simulink model "LDPC_Decoder_Ex1"  (R2024a)
settings: Solver=VariableStepAuto  StartTime=0.0  StopTime=64800+64800  RelTol=1e-3
undefined symbols (not defined in the file or in its folder): Configured, DVB, es1, F, Initialized_retain_I, Pre, S, S2, vsva2488, X, xcvr1602
libraries: hdlBasic x37, dspsrcs4 x3, hdlDSPIP x1, vmcUtilities x1
settings Model: Creator=nanumolu  LastModifiedBy=sdegala
settings ConfigComp: CovBoundaryAbsTol=1.0e-5

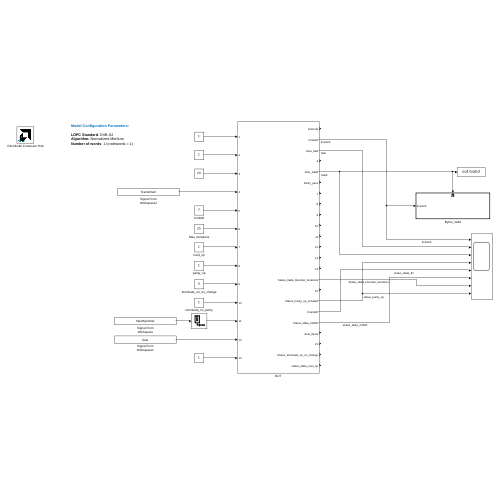
[thumbnail: Simulink's stored preview of the top-level diagram]
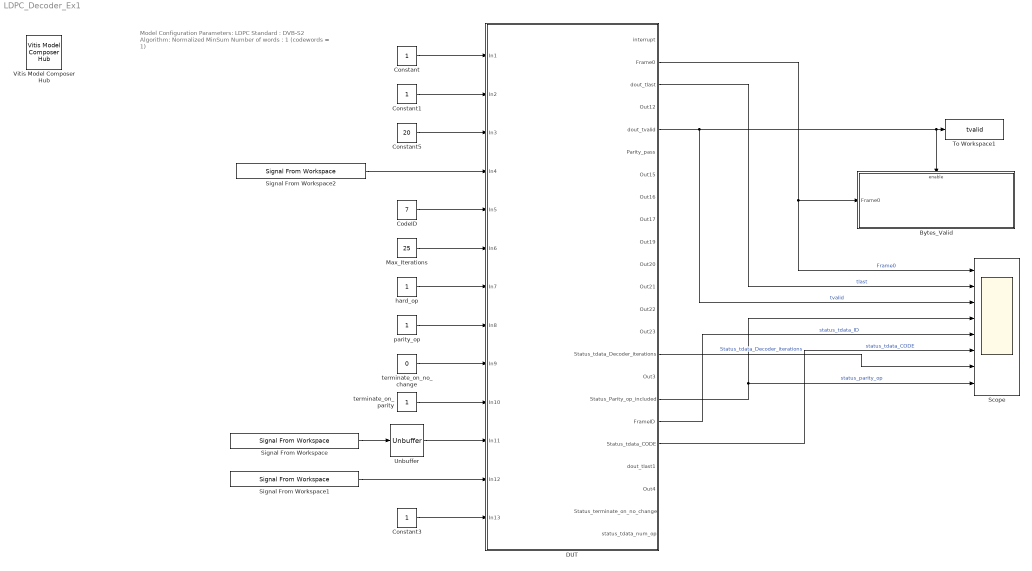
== system LDPC_Decoder_Ex1 ==
  note: Model Configuration Parameters:
      |
      | LDPC Standard : DVB-S2
      | Algorithm: Normalized MinSum
      | Number of words : 1 (codewords = 1)
  Bytes_Valid : Subsystem
  CodeID : Constant  Value=7  SampleTime=1
  Constant : Constant  SampleTime=1
  Constant1 : Constant  SampleTime=1
  Constant3 : Constant  SampleTime=1
  Constant5 : Constant  Value=20  SampleTime=1
  DUT : Subsystem
  Max_Iterations : Constant  Value=25  SampleTime=1
  Scope : Scope  NumInputPorts=8
  Signal From Workspace : dspsrcs4/Signal From Workspace  X=InputSymbols  Ts=1  nsamps=64800  OutputAfterFinalValue=Setting to zero  ignoreOrWarnInputAndFrameLengths=off  OutputFrames=off
  Signal From Workspace1 : dspsrcs4/Signal From Workspace  X=tlast  Ts=1  nsamps=1  OutputAfterFinalValue=Setting to zero  ignoreOrWarnInputAndFrameLengths=off  OutputFrames=off
  Signal From Workspace2 : dspsrcs4/Signal From Workspace  X=FrameNum  Ts=1  nsamps=1  OutputAfterFinalValue=Setting to zero  ignoreOrWarnInputAndFrameLengths=off  OutputFrames=off
  To Workspace1 : ToWorkspace  VariableName=tvalid  SampleTime=-1
      settings: Save2DSignal=2-D array (concatenate along first dimension)
  Unbuffer : Unbuffer
  Vitis Model Composer Hub : vmcUtilities/Vitis Model Composer Hub  Tag=genX  CodeGeneration=off  SubsystemName=DUT  BlockHierPath=Channalizer_smoke  CompilationType=HDLCompilation  SubsystemType=HDLNode  ExportTypeV2=HDL Netlist  StartColumn=1  NumberOfColumns=1  TargetDirectory=./netlist_chan_vlg  exportDesign=on  analyzeDesign=off  validateDesignOnHw=off  ExportType=AI Engines  IpVendor=xilinx.com  IpLibrary=hls  IpVersion=1.0  IpHWLanguage=Verilog  AieCompilerOptions={}  AieSimulatorOptions={}  CreateTestbench=on  TestbenchStackSize=10  RunRtlSim=off  RunCSim=off  RunAieSim=off  AieSimTimeout=50000  RunAieSimProfiling=off  LaunchVitisAnalyzer=off  PlotOutput=off  RunX86Sim=off  X86SimTimeout=10  GenHwImage=off  GenLibadfXo=on  GenHwValidationCode=off  PlatformType=Not Specified  HwSystemType=Baremetal  HwValidationTarget=hw  ProjDevice=xcvr1602-vsva2488-2MP-e-S-es1  ProjDevicePart=xcvr1602-vsva2488-2MP-e-S-es1  AIEType=AIE  SamplePeriod=-1  ClockFrequency=200  DataPathParallelism=1  xilinxfamily=versalairfes1  part=xcvr1602  speed=-2MP-e-S-es1  package=vsva2488  directory=./netlist/ip/DUT/src  testbench=off  incr_netlist=off  synthesis_tool=Vivado  clock_wrapper=Clock Enables  dbl_ovrd=According to Block Masks  dcm_input_clock_period=10  sysclk_period=10  simulink_period=1  eval_field=0  IPInfoJsonString="{\"DUTSubsystemName\":\"Channalizer_smoke\",\"HDLSubsystem\":{\"SubsystemName\":\"Channalizer_smoke\",\"IPName\":\"Copy_of_hamilton_vrf_fft\",\"IPLibrary\":\"VMC\",\"IPVendor\":\"User Company\",\"IPVersion\":\"1.0\",\"TargetDirectory\":\"./netlist_chan_vlg\",\"SubsystemDir\":\"./netlist_chan_vlg/ip/Channalizer_smoke\",\"FreqHz\":\"100000000\"},\"SubsystemTag\":\"HDLNode\"}"  LogFileName=/proj/dsv_xhd/ravalib/Head/Tests/REL/2025.1/dsv/modelcomposer/hdl/regression/channelizer/smoke/netlist_chan_vlg/model_composer.log  NThreads=4  IPConfigFile=/tmp/vmctmp-10364637636032824832/Channalizer_smoke_ipconfig.json
  hard_op : Constant  SampleTime=1
  parity_op : Constant  SampleTime=1
  terminate_on_no_change : Constant  Value=0  SampleTime=1
  terminate_on_parity : Constant  SampleTime=1
  wires:
  Constant/1 -> DUT/1(In1)
  Constant1/1 -> DUT/2(In2)
  Constant5/1 -> DUT/3(In3)
  Signal From Workspace2/1 -> DUT/4(In4)
  CodeID/1 -> DUT/5(In5)
  Max_Iterations/1 -> DUT/6(In6)
  hard_op/1 -> DUT/7(In7)
  parity_op/1 -> DUT/8(In8)
  terminate_on_no_change/1 -> DUT/9(In9)
  terminate_on_parity/1 -> DUT/10(In10)
  Constant3/1 -> DUT/13(In13)
  Signal From Workspace1/1 -> DUT/12(In12)
  DUT/2(Frame0) -> Scope/1, Bytes_Valid/1(Frame0)  "Frame0"
  DUT/5(dout_tvalid) -> To Workspace1/1, Bytes_Valid/Enable, Scope/3  "tvalid"
  DUT/3(dout_tlast) -> Scope/2  "tlast"
  DUT/17(Status_Parity_op_included) -> Scope/4, Scope/8  "status_parity_op"
  DUT/18(FrameID) -> Scope/5  "status_tdata_ID"
  DUT/19(Status_tdata_CODE) -> Scope/6  "status_tdata_CODE"
  Signal From Workspace/1 -> Unbuffer/1
  Unbuffer/1 -> DUT/11(In11)
  DUT/15(Status_tdata_Decoder_iterations) -> Scope/7  "Status_tdata_Decoder_iterations"

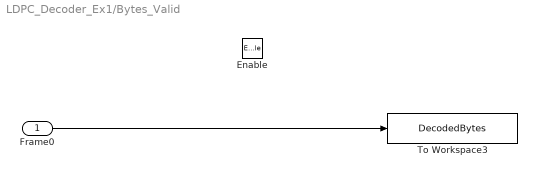
== system LDPC_Decoder_Ex1/Bytes_Valid ==
  Frame0 : Inport
  Enable : EnablePort
  To Workspace3 : ToWorkspace  VariableName=DecodedBytes  SampleTime=-1
      settings: Save2DSignal=2-D array (concatenate along first dimension)
  wires:
  Frame0/1 -> To Workspace3/1

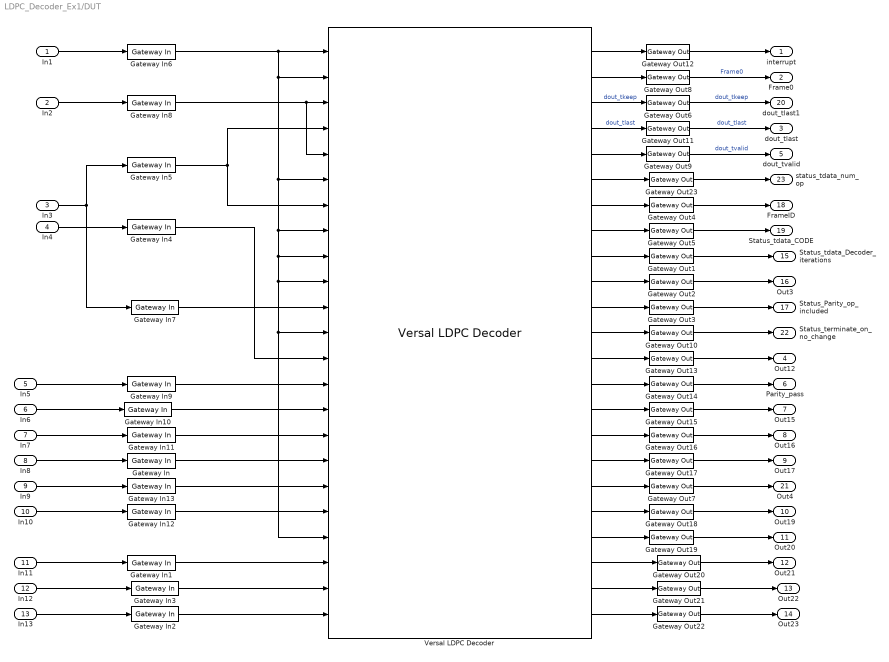
== system LDPC_Decoder_Ex1/DUT ==
  In1 : Inport
  In2 : Inport  Port=2
  In3 : Inport  Port=3
  In4 : Inport  Port=4
  In5 : Inport  Port=5
  In6 : Inport  Port=6
  In7 : Inport  Port=7
  In8 : Inport  Port=8
  In9 : Inport  Port=9
  In10 : Inport  Port=10
  In11 : Inport  Port=11
  In12 : Inport  Port=12
  In13 : Inport  Port=13
  Gateway In{,11..13} (4 alike) : hdlBasic/Gateway In  gui_display_data_type=Fixed-point  arith_type=Unsigned  n_bits=1  bin_pt=0  preci_type=Single  exp_width=8  frac_width=24  rows=1  columns=1  quantization="Round  (unbiased: +/- Inf)"  overflow=Saturate  period=1  UseAsADC=off  ADCChannel='1'  interface=None  automatic_assignment=on  address_offset=hex2dec('00')  intf_name=''  intf_description=''  default_value=0  timing_constraint=None  locs_specified=off  LOCs={}  io_standard={}  inherit_from_input=off  hdl_port=on  XmcBlockStatus=1  maskContainerNames=group4  block_type=gatewayin  block_config=sysgen:gateway_in_config  block_width_w=590  block_height_w=620  block_width=640  block_height=850
  Gateway In1 : hdlBasic/Gateway In  gui_display_data_type=Fixed-point  arith_type=Signed (2's comp)  n_bits=8  bin_pt=2  preci_type=Single  exp_width=8  frac_width=24  rows=1  columns=1  quantization="Round  (unbiased: +/- Inf)"  overflow=Saturate  period=1  UseAsADC=off  ADCChannel='1'  interface=None  automatic_assignment=on  address_offset=hex2dec('00')  intf_name=''  intf_description=''  default_value=0  timing_constraint=None  locs_specified=off  LOCs={}  io_standard={}  inherit_from_input=off  hdl_port=on  XmcBlockStatus=1  maskContainerNames=group4  block_type=gatewayin  block_config=sysgen:gateway_in_config  block_width_w=590  block_height_w=620  block_width=640  block_height=850
  Gateway In10 : hdlBasic/Gateway In  gui_display_data_type=Fixed-point  arith_type=Unsigned  n_bits=6  bin_pt=0  preci_type=Single  exp_width=8  frac_width=24  rows=1  columns=1  quantization="Round  (unbiased: +/- Inf)"  overflow=Saturate  period=1  UseAsADC=off  ADCChannel='1'  interface=None  automatic_assignment=on  address_offset=hex2dec('00')  intf_name=''  intf_description=''  default_value=0  timing_constraint=None  locs_specified=off  LOCs={}  io_standard={}  inherit_from_input=off  hdl_port=on  XmcBlockStatus=1  maskContainerNames=group4  block_type=gatewayin  block_config=sysgen:gateway_in_config  block_width_w=590  block_height_w=620  block_width=640  block_height=850
  Gateway In2 : hdlBasic/Gateway In  gui_display_data_type=Boolean  arith_type=Boolean  n_bits=1  bin_pt=0  preci_type=Single  exp_width=8  frac_width=24  rows=1  columns=1  quantization="Round  (unbiased: +/- Inf)"  overflow=Saturate  period=1  UseAsADC=off  ADCChannel='1'  interface=None  automatic_assignment=on  address_offset=hex2dec('00')  intf_name=''  intf_description=''  default_value=0  timing_constraint=None  locs_specified=off  LOCs={}  io_standard={}  inherit_from_input=off  hdl_port=on  XmcBlockStatus=1  maskContainerNames=group4  block_type=gatewayin  block_config=sysgen:gateway_in_config  block_width_w=590  block_height_w=620  block_width=640  block_height=850
  Gateway In3 : hdlBasic/Gateway In  gui_display_data_type=Boolean  arith_type=Boolean  n_bits=1  bin_pt=0  preci_type=Single  exp_width=8  frac_width=24  rows=1  columns=1  quantization="Round  (unbiased: +/- Inf)"  overflow=Saturate  period=1  UseAsADC=off  ADCChannel='1'  interface=None  automatic_assignment=on  address_offset=hex2dec('00')  intf_name=''  intf_description=''  default_value=0  timing_constraint=None  locs_specified=off  LOCs={}  io_standard={}  inherit_from_input=off  hdl_port=on  XmcBlockStatus=1  maskContainerNames=group4  block_type=gatewayin  block_config=sysgen:gateway_in_config  block_width_w=590  block_height_w=620  block_width=640  block_height=850
  Gateway In4 : hdlBasic/Gateway In  gui_display_data_type=Fixed-point  arith_type=Unsigned  n_bits=8  bin_pt=0  preci_type=Single  exp_width=8  frac_width=24  rows=1  columns=1  quantization="Round  (unbiased: +/- Inf)"  overflow=Saturate  period=1  UseAsADC=off  ADCChannel='1'  interface=None  automatic_assignment=on  address_offset=hex2dec('00')  intf_name=''  intf_description=''  default_value=0  timing_constraint=None  locs_specified=off  LOCs={}  io_standard={}  inherit_from_input=off  hdl_port=on  XmcBlockStatus=1  maskContainerNames=group4  block_type=gatewayin  block_config=sysgen:gateway_in_config  block_width_w=590  block_height_w=620  block_width=640  block_height=850
  Gateway In5 : hdlBasic/Gateway In  gui_display_data_type=Fixed-point  arith_type=Signed (2's comp)  n_bits=18  bin_pt=0  preci_type=Single  exp_width=8  frac_width=24  rows=1  columns=1  quantization="Round  (unbiased: +/- Inf)"  overflow=Saturate  period=1  UseAsADC=off  ADCChannel='1'  interface=None  automatic_assignment=on  address_offset=hex2dec('00')  intf_name=''  intf_description=''  default_value=0  timing_constraint=None  locs_specified=off  LOCs={}  io_standard={}  inherit_from_input=off  hdl_port=on  XmcBlockStatus=1  maskContainerNames=group4  block_type=gatewayin  block_config=sysgen:gateway_in_config  block_width_w=590  block_height_w=620  block_width=640  block_height=850
  Gateway In6 : hdlBasic/Gateway In  gui_display_data_type=Boolean  arith_type=Boolean  n_bits=16  bin_pt=14  preci_type=Single  exp_width=8  frac_width=24  rows=1  columns=1  quantization="Round  (unbiased: +/- Inf)"  overflow=Saturate  period=1  UseAsADC=off  ADCChannel='1'  interface=None  automatic_assignment=on  address_offset=hex2dec('00')  intf_name=''  intf_description=''  default_value=0  timing_constraint=None  locs_specified=off  LOCs={}  io_standard={}  inherit_from_input=off  hdl_port=on  XmcBlockStatus=1  maskContainerNames=group4  block_type=gatewayin  block_config=sysgen:gateway_in_config  block_width_w=590  block_height_w=620  block_width=640  block_height=850
  Gateway In7 : hdlBasic/Gateway In  gui_display_data_type=Fixed-point  arith_type=Signed (2's comp)  n_bits=32  bin_pt=0  preci_type=Single  exp_width=8  frac_width=24  rows=1  columns=1  quantization="Round  (unbiased: +/- Inf)"  overflow=Saturate  period=1  UseAsADC=off  ADCChannel='1'  interface=None  automatic_assignment=on  address_offset=hex2dec('00')  intf_name=''  intf_description=''  default_value=0  timing_constraint=None  locs_specified=off  LOCs={}  io_standard={}  inherit_from_input=off  hdl_port=on  XmcBlockStatus=1  maskContainerNames=group4  block_type=gatewayin  block_config=sysgen:gateway_in_config  block_width_w=590  block_height_w=620  block_width=640  block_height=850
  Gateway In8 : hdlBasic/Gateway In  gui_display_data_type=Boolean  arith_type=Boolean  n_bits=16  bin_pt=14  preci_type=Single  exp_width=8  frac_width=24  rows=1  columns=1  quantization="Round  (unbiased: +/- Inf)"  overflow=Saturate  period=1  UseAsADC=off  ADCChannel='1'  interface=None  automatic_assignment=on  address_offset=hex2dec('00')  intf_name=''  intf_description=''  default_value=0  timing_constraint=None  locs_specified=off  LOCs={}  io_standard={}  inherit_from_input=off  hdl_port=on  XmcBlockStatus=1  maskContainerNames=group4  block_type=gatewayin  block_config=sysgen:gateway_in_config  block_width_w=590  block_height_w=620  block_width=640  block_height=850
  Gateway In9 : hdlBasic/Gateway In  gui_display_data_type=Fixed-point  arith_type=Unsigned  n_bits=7  bin_pt=0  preci_type=Single  exp_width=8  frac_width=24  rows=1  columns=1  quantization="Round  (unbiased: +/- Inf)"  overflow=Saturate  period=1  UseAsADC=off  ADCChannel='1'  interface=None  automatic_assignment=on  address_offset=hex2dec('00')  intf_name=''  intf_description=''  default_value=0  timing_constraint=None  locs_specified=off  LOCs={}  io_standard={}  inherit_from_input=off  hdl_port=on  XmcBlockStatus=1  maskContainerNames=group4  block_type=gatewayin  block_config=sysgen:gateway_in_config  block_width_w=590  block_height_w=620  block_width=640  block_height=850
  Gateway Out{1..7,9..23} (22 alike) : hdlBasic/Gateway Out  inherit_from_input=off  bool_to_boolean=off  hdl_port=on  rows=1  columns=1  UseAsDAC=off  DACChannel='1'  interface=None  automatic_assignment=on  address_offset=hex2dec('00')  intf_name=''  intf_description=''  timing_constraint=None  locs_specified=off  LOCs={}  io_standard={}  XmcBlockStatus=1  maskContainerNames=group4  block_type=gatewayout  block_config=sysgen:gateway_out_config  block_width_w=590  block_height_w=620  block_width=620  block_height=750
  Gateway Out8 : hdlBasic/Gateway Out  inherit_from_input=on  bool_to_boolean=off  hdl_port=on  rows=1  columns=1  UseAsDAC=off  DACChannel='1'  interface=None  automatic_assignment=on  address_offset=hex2dec('00')  intf_name=''  intf_description=''  timing_constraint=None  locs_specified=off  LOCs={}  io_standard={}  XmcBlockStatus=1  maskContainerNames=group4  block_type=gatewayout  block_config=sysgen:gateway_out_config  block_width_w=590  block_height_w=620  block_width=620  block_height=750
  Versal LDPC Decoder : hdlDSPIP/Versal LDPC Decoder  standard=DVB-S2(X)  ldpc_decode_algorithm_source=Initialized  ldpc_decode_algorithm_modifier_source=Initialized  ldpc_decode_sat_bits_source=Initialized  ldpc_decode_max_schedule_source=Initialized  ldpc_decode_code_definition='no_file_loaded'  ldpc_decode_overrides=on  ldpc_decode_algorithm=Normalized_MinSum  ldpc_decode_algorithm_modifier=1  ldpc_decode_sat_bits=6B  ldpc_decode_max_schedule=0  parameter_interface=Initialized_retain_I/F  enable_ifs=on  Interrupts=on  ecc_interrupts=None  bypass=off  din_interface=Pre-Configured  din_lanes=1  din_words_configuration=Fixed  din_words=1  dout_interface=Pre-Configured  dout_lanes=1  dout_words_configuration=Fixed  dout_words=1  throughput_utilization=100  ip_name=Versal LDPC Decoder  ip_version=1.0  dsptool_ready=false  ipcore_usecache=true  ipcore_useipmodelcache=true  wrapper_available=true  port_translation_map={ 'aclken' => 'en', aresetn' => 'rst' }  structural_sim=true  ipcore_do_not_force_period=true  XmcBlockStatus=1  maskContainerNames=tabcontainer1  block_type=versal_ldpc_v1_0  block_config=sysgen:rodinimport_config
  interrupt : Outport
  Frame0 : Outport  Port=2
  dout_tlast : Outport  Port=3
  Out12 : Outport  Port=4
  dout_tvalid : Outport  Port=5
  Parity_pass : Outport  Port=6
  Out15 : Outport  Port=7
  Out16 : Outport  Port=8
  Out17 : Outport  Port=9
  Out19 : Outport  Port=10
  Out20 : Outport  Port=11
  Out21 : Outport  Port=12
  Out22 : Outport  Port=13
  Out23 : Outport  Port=14
  Status_tdata_Decoder_iterations : Outport  Port=15
  Out3 : Outport  Port=16
  Status_Parity_op_included : Outport  Port=17
  FrameID : Outport  Port=18
  Status_tdata_CODE : Outport  Port=19
  dout_tlast1 : Outport  Port=20
  Out4 : Outport  Port=21
  Status_terminate_on_no_change : Outport  Port=22
  status_tdata_num_op : Outport  Port=23
  wires:
  Versal LDPC Decoder/1 -> Gateway Out12/1
  Gateway In12/1 -> Versal LDPC Decoder/19
  Gateway In/1 -> Versal LDPC Decoder/17
  Gateway In11/1 -> Versal LDPC Decoder/16
  Gateway In9/1 -> Versal LDPC Decoder/14
  Versal LDPC Decoder/15 -> Gateway Out15/1
  Gateway Out9/1 -> dout_tvalid/1  "dout_tvalid"
  Gateway In7/1 -> Versal LDPC Decoder/11
  Gateway In6/1 -> Versal LDPC Decoder/6, Versal LDPC Decoder/8, Versal LDPC Decoder/9, Versal LDPC Decoder/10, Versal LDPC Decoder/12, Versal LDPC Decoder/20, Versal LDPC Decoder/2, Versal LDPC Decoder/1
  Versal LDPC Decoder/17 -> Gateway Out17/1
  In5/1 -> Gateway In9/1
  Gateway In5/1 -> Versal LDPC Decoder/7, Versal LDPC Decoder/4
  Gateway In2/1 -> Versal LDPC Decoder/23
  Versal LDPC Decoder/19 -> Gateway Out18/1
  Versal LDPC Decoder/20 -> Gateway Out19/1
  Gateway In4/1 -> Versal LDPC Decoder/13
  In3/1 -> Gateway In7/1, Gateway In5/1
  Versal LDPC Decoder/4 -> Gateway Out11/1  "dout_tlast"
  In13/1 -> Gateway In2/1
  In6/1 -> Gateway In10/1
  In7/1 -> Gateway In11/1
  In4/1 -> Gateway In4/1
  Gateway Out8/1 -> Frame0/1  "Frame0"
  In1/1 -> Gateway In6/1
  Versal LDPC Decoder/21 -> Gateway Out20/1
  In11/1 -> Gateway In1/1
  In8/1 -> Gateway In/1
  In10/1 -> Gateway In12/1
  In9/1 -> Gateway In13/1
  Gateway In3/1 -> Versal LDPC Decoder/22
  Versal LDPC Decoder/13 -> Gateway Out13/1
  Gateway In13/1 -> Versal LDPC Decoder/18
  In2/1 -> Gateway In8/1
  Versal LDPC Decoder/14 -> Gateway Out14/1
  Versal LDPC Decoder/16 -> Gateway Out16/1
  Versal LDPC Decoder/23 -> Gateway Out22/1
  Gateway In10/1 -> Versal LDPC Decoder/15
  Gateway In8/1 -> Versal LDPC Decoder/3, Versal LDPC Decoder/5
  In12/1 -> Gateway In3/1
  Versal LDPC Decoder/22 -> Gateway Out21/1
  Gateway Out11/1 -> dout_tlast/1  "dout_tlast"
  Gateway Out12/1 -> interrupt/1
  Gateway Out13/1 -> Out12/1
  Gateway Out14/1 -> Parity_pass/1
  Gateway Out15/1 -> Out15/1
  Gateway Out16/1 -> Out16/1
  Gateway Out17/1 -> Out17/1
  Gateway Out18/1 -> Out19/1
  Gateway Out19/1 -> Out20/1
  Gateway Out20/1 -> Out21/1
  Gateway Out21/1 -> Out22/1
  Gateway Out22/1 -> Out23/1
  Gateway In1/1 -> Versal LDPC Decoder/21
  Versal LDPC Decoder/5 -> Gateway Out9/1
  Versal LDPC Decoder/2 -> Gateway Out8/1
  Gateway Out1/1 -> Status_tdata_Decoder_iterations/1
  Versal LDPC Decoder/9 -> Gateway Out1/1
  Versal LDPC Decoder/10 -> Gateway Out2/1
  Gateway Out2/1 -> Out3/1
  Versal LDPC Decoder/11 -> Gateway Out3/1
  Gateway Out3/1 -> Status_Parity_op_included/1
  Gateway Out4/1 -> FrameID/1
  Versal LDPC Decoder/7 -> Gateway Out4/1
  Versal LDPC Decoder/8 -> Gateway Out5/1
  Gateway Out5/1 -> Status_tdata_CODE/1
  Gateway Out6/1 -> dout_tlast1/1  "dout_tkeep"
  Versal LDPC Decoder/3 -> Gateway Out6/1  "dout_tkeep"
  Gateway Out7/1 -> Out4/1
  Versal LDPC Decoder/18 -> Gateway Out7/1
  Gateway Out10/1 -> Status_terminate_on_no_change/1
  Versal LDPC Decoder/12 -> Gateway Out10/1
  Gateway Out23/1 -> status_tdata_num_op/1
  Versal LDPC Decoder/6 -> Gateway Out23/1
